simulink model "ex6_1"  (R2024b)
settings: Solver=VariableStepAuto  StartTime=0.0  StopTime=10.0  RelTol=1e-3
libraries: simulink x1
settings Model: Creator=pc  LastModifiedBy=pc

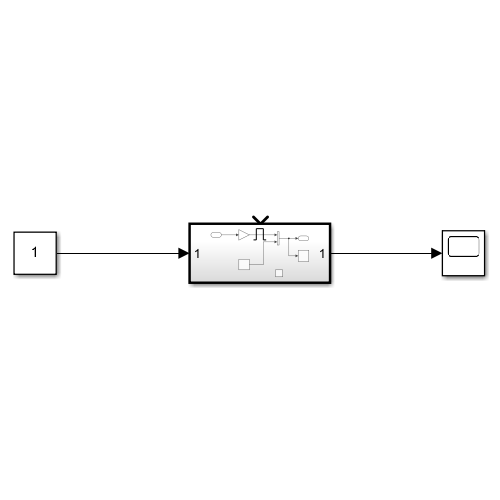
[thumbnail: Simulink's stored preview of the top-level diagram]
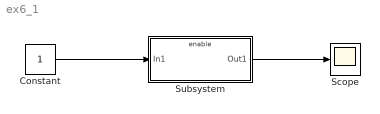
== system ex6_1 ==
  Constant : Constant
  Scope : Scope
  Subsystem : Subsystem
  wires:
  Constant/1 -> Subsystem/1(In1)
  Subsystem/1(Out1) -> Scope/1

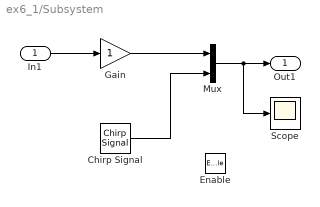
== system ex6_1/Subsystem ==
  In1 : Inport
  Enable : EnablePort
  Chirp Signal : simulink/Sources/Chirp Signal  f1=0.1  T=100  f2=1
  Gain : Gain
  Mux : Mux  Inputs=2
  Scope : Scope
  Out1 : Outport
  wires:
  In1/1 -> Gain/1
  Chirp Signal/1 -> Mux/2
  Gain/1 -> Mux/1
  Mux/1 -> Out1/1, Scope/1
